simulink model "HydroPowertest2"  (R2024b)
settings: Solver=FixedStepAuto  StartTime=0.0  StopTime=10  FixedStep=0.0001  RelTol=1e-3
values from neighbouring files (symbols this model uses):
  A1 = [-Rs/Ld 0 ;0 -Rs/Lq ]    [Generator_Data.m]
  A2 = [0 Lq/Ld ;-Ld/Lq 0]    [Generator_Data.m]
  B1 = [-1/Ld 0 0;0 -1/Lq 0]    [Generator_Data.m]
  B2 = [0 0 0;0  0 1/Lq]    [Generator_Data.m]
  Ld = 1.4e-3+L_charge    (= 0.0014)    [Generator_Data.m]    (also in Generator_Datatest.m = 0.0231)
  Lq = 2.8e-3+L_charge    (= 0.0028)    [Generator_Data.m]    (also in Generator_Datatest.m = 0.0231)
  P = 4    [Generator_Data.m]    (also in Generator_Datatest.m = 3)
  Phif = 0.8    [Generator_Data.m]
  Rs = 0.6+R_charge    (= 0.6)    [Generator_Data.m]    (also in Generator_Datatest.m = 0.48)
  wm = 2*pi*50/P    (= 78.5398163397)    [Generator_Data.m]
settings Model: Creator=belka  LastModifiedBy=Nasser
settings DebuggingCC: SignalResolutionControl=TryResolveAll
settings RTWCC: GPUComputeCapability=3.5

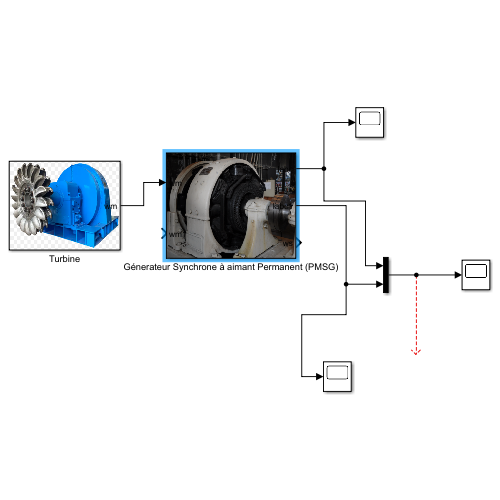
[thumbnail: Simulink's stored preview of the top-level diagram]
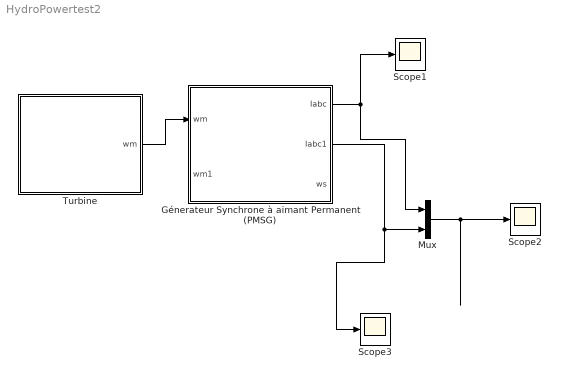
== system HydroPowertest2 ==
  Génerateur Synchrone à aimant Permanent (PMSG) : Subsystem
      mask Display: image('generateur.png');
  Mux : Mux  Inputs=2
  Scope1 : Scope
  Scope2 : Scope
  Scope3 : Scope
  Turbine : Subsystem
      mask Display: image('turbine.png');
  wires:
  Génerateur Synchrone à aimant Permanent (PMSG)/1(Iabc) -> Scope1/1, Mux/1
  Turbine/1(wm) -> Génerateur Synchrone à aimant Permanent (PMSG)/1(wm)
  Mux/1 -> Scope2/1
  Génerateur Synchrone à aimant Permanent (PMSG)/2(Iabc1) -> Scope3/1, Mux/2

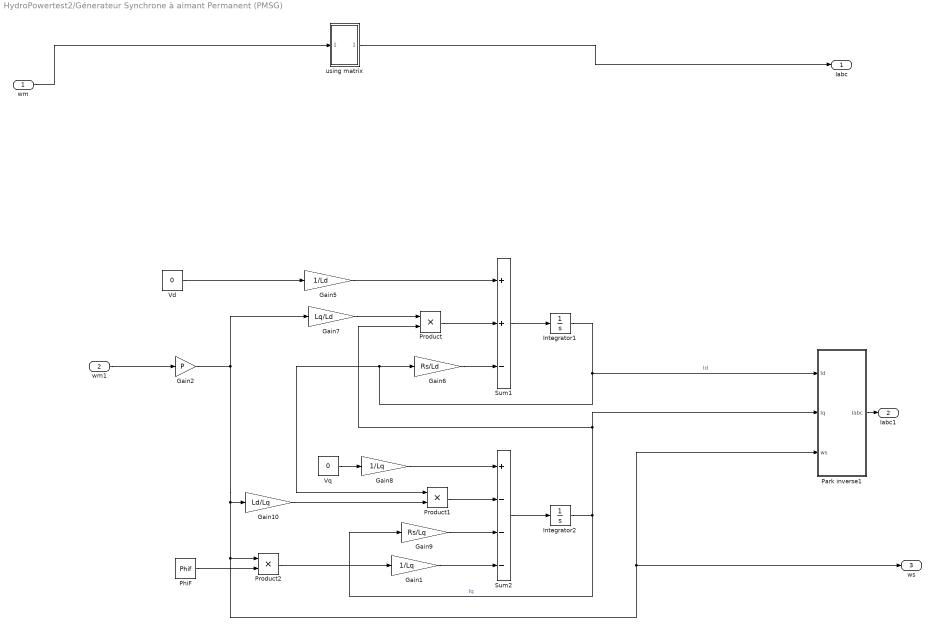
== system HydroPowertest2/Génerateur Synchrone à aimant Permanent (PMSG) ==
  wm : Inport
  wm1 : Inport  Port=2
  Gain1 : Gain  Gain=1/Lq
  Gain10 : Gain  Gain=Ld/Lq
  Gain2 : Gain  Gain=P
  Gain5 : Gain  Gain=1/Ld
  Gain6 : Gain  Gain=Rs/Ld
  Gain7 : Gain  Gain=Lq/Ld
  Gain8 : Gain  Gain=1/Lq
  Gain9 : Gain  Gain=Rs/Lq
  Integrator1 : Integrator
  Integrator2 : Integrator
  Park inverse1 : Subsystem
      mask Display: disp('Park\n Inverse')
  PhiF : Constant  Value=Phif
  Product : Product
  Product1 : Product
  Product2 : Product
  Sum1 : Sum  Inputs=++-
  Sum2 : Sum  Inputs=+---
  Vd : Constant  Value=0
  Vq : Constant  Value=0
  using matrix : Subsystem
  Iabc : Outport
  Iabc1 : Outport  Port=2
  ws : Outport  Port=3
  wires:
  wm/1 -> using matrix/1(In1)
  Park inverse1/1(Iabc) -> Iabc1/1
  using matrix/1(Iabc) -> Iabc/1
  Gain6/1 -> Sum1/3
  Vd/1 -> Gain5/1
  Gain5/1 -> Sum1/1
  Integrator2/1 -> Park inverse1/2(Iq), Product/2, Gain9/1  "Iq"
  Sum1/1 -> Integrator1/1
  Sum2/1 -> Integrator2/1
  Vq/1 -> Gain8/1
  Gain8/1 -> Sum2/1
  Integrator1/1 -> Park inverse1/1(Id), Gain6/1, Product1/1  "Id"
  Gain10/1 -> Product1/2
  Gain9/1 -> Sum2/3
  PhiF/1 -> Product2/2
  Product2/1 -> Gain1/1
  Product/1 -> Sum1/2
  Gain1/1 -> Sum2/4
  Product1/1 -> Sum2/2
  wm1/1 -> Gain2/1
  Gain2/1 -> Park inverse1/3(ws), ws/1, Product2/1, Gain10/1, Gain7/1
  Gain7/1 -> Product/1

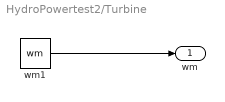
== system HydroPowertest2/Turbine ==
  wm1 : Constant  Value=wm
  wm : Outport
  wires:
  wm1/1 -> wm/1

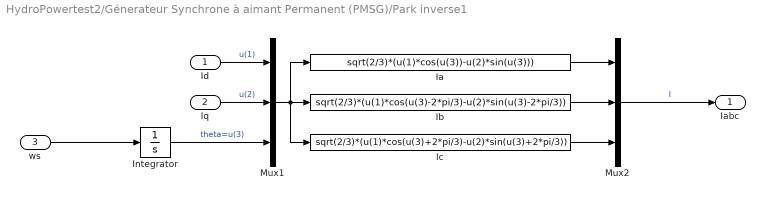
== system HydroPowertest2/Génerateur Synchrone à aimant Permanent (PMSG)/Park inverse1 ==
  Id : Inport
  Iq : Inport  Port=2
  ws : Inport  Port=3
  Ia : Fcn  Expr=sqrt(2/3)*(u(1)*cos(u(3))-u(2)*sin(u(3)))
  Ib : Fcn  Expr=sqrt(2/3)*(u(1)*cos(u(3)-2*pi/3)-u(2)*sin(u(3)-2*pi/3))
  Ic : Fcn  Expr=sqrt(2/3)*(u(1)*cos(u(3)+2*pi/3)-u(2)*sin(u(3)+2*pi/3))
  Integrator : Integrator
  Mux1 : Mux  Inputs=3
  Mux2 : Mux  Inputs=3
  Iabc : Outport
  wires:
  ws/1 -> Integrator/1
  Integrator/1 -> Mux1/3  "theta=u(3)"
  Id/1 -> Mux1/1  "u(1)"
  Iq/1 -> Mux1/2  "u(2)"
  Ia/1 -> Mux2/1
  Ic/1 -> Mux2/3
  Ib/1 -> Mux2/2
  Mux2/1 -> Iabc/1  "I"
  Mux1/1 -> Ia/1, Ic/1, Ib/1

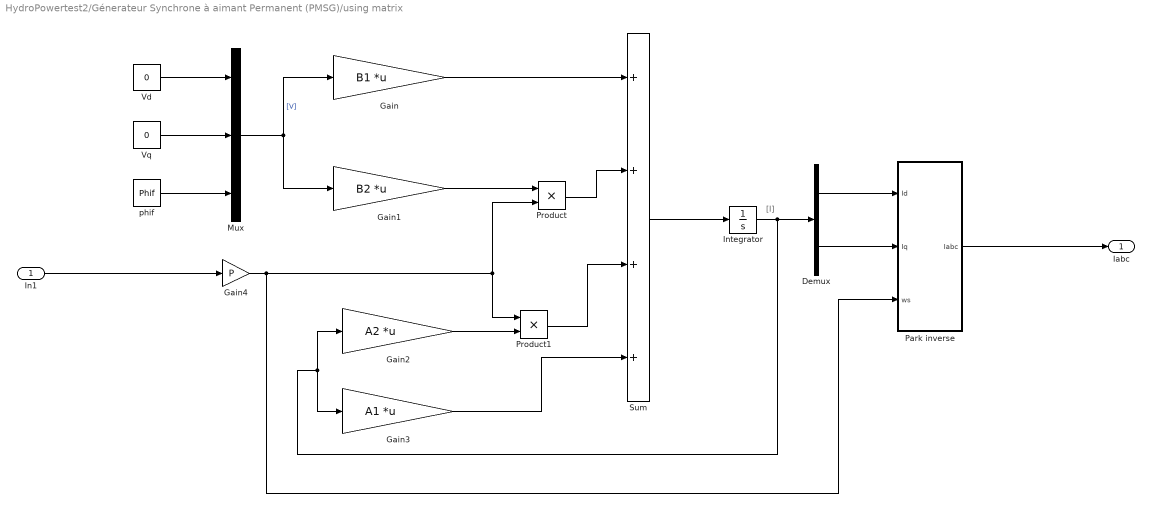
== system HydroPowertest2/Génerateur Synchrone à aimant Permanent (PMSG)/using matrix ==
  note: [I]
  In1 : Inport
  Demux : Demux  Outputs=2
  Gain : Gain  Gain=B1  Multiplication=Matrix(K*u)
  Gain1 : Gain  Gain=B2  Multiplication=Matrix(K*u)
  Gain2 : Gain  Gain=A2  Multiplication=Matrix(K*u)
  Gain3 : Gain  Gain=A1  Multiplication=Matrix(K*u)
  Gain4 : Gain  Gain=P
  Integrator : Integrator
  Mux : Mux  Inputs=3
  Park inverse : Subsystem
      mask Display: disp('Park\n Inverse')
  Product : Product
  Product1 : Product
  Sum : Sum  Inputs=++++
  Vd : Constant  Value=0
  Vq : Constant  Value=0
  phif : Constant  Value=Phif
  Iabc : Outport
  wires:
  phif/1 -> Mux/3
  Product/1 -> Sum/2
  Gain4/1 -> Park inverse/3(ws), Product1/1, Product/2
  Gain2/1 -> Product1/2
  Demux/1 -> Park inverse/1(Id)
  Sum/1 -> Integrator/1
  Mux/1 -> Gain1/1, Gain/1  "[V]"
  Park inverse/1(Iabc) -> Iabc/1
  Gain/1 -> Sum/1
  Vq/1 -> Mux/2
  Vd/1 -> Mux/1
  Integrator/1 -> Demux/1, Gain3/1, Gain2/1
  Gain1/1 -> Product/1
  Product1/1 -> Sum/3
  Demux/2 -> Park inverse/2(Iq)
  Gain3/1 -> Sum/4
  In1/1 -> Gain4/1

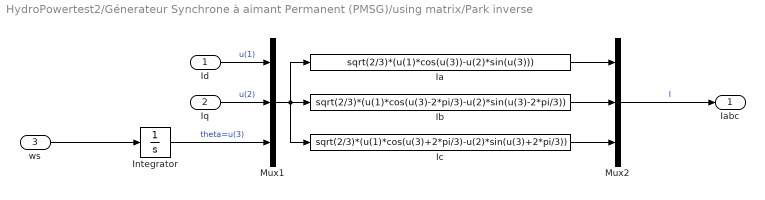
== system HydroPowertest2/Génerateur Synchrone à aimant Permanent (PMSG)/using matrix/Park inverse ==
  Id : Inport
  Iq : Inport  Port=2
  ws : Inport  Port=3
  Ia : Fcn  Expr=sqrt(2/3)*(u(1)*cos(u(3))-u(2)*sin(u(3)))
  Ib : Fcn  Expr=sqrt(2/3)*(u(1)*cos(u(3)-2*pi/3)-u(2)*sin(u(3)-2*pi/3))
  Ic : Fcn  Expr=sqrt(2/3)*(u(1)*cos(u(3)+2*pi/3)-u(2)*sin(u(3)+2*pi/3))
  Integrator : Integrator
  Mux1 : Mux  Inputs=3
  Mux2 : Mux  Inputs=3
  Iabc : Outport
  wires:
  Mux1/1 -> Ib/1, Ic/1, Ia/1
  Mux2/1 -> Iabc/1  "I"
  Ib/1 -> Mux2/2
  Ic/1 -> Mux2/3
  Ia/1 -> Mux2/1
  Iq/1 -> Mux1/2  "u(2)"
  Id/1 -> Mux1/1  "u(1)"
  Integrator/1 -> Mux1/3  "theta=u(3)"
  ws/1 -> Integrator/1
